simulink model "Q2"  (R2018a)
settings: Solver=VariableStepDiscrete  StartTime=0.0  StopTime=10  RelTol=1e-3
libraries: powerlib x10
settings Model: Creator=enes_  LastModifiedBy=nailt
settings CodeAppCC: StateflowObjectComments=on

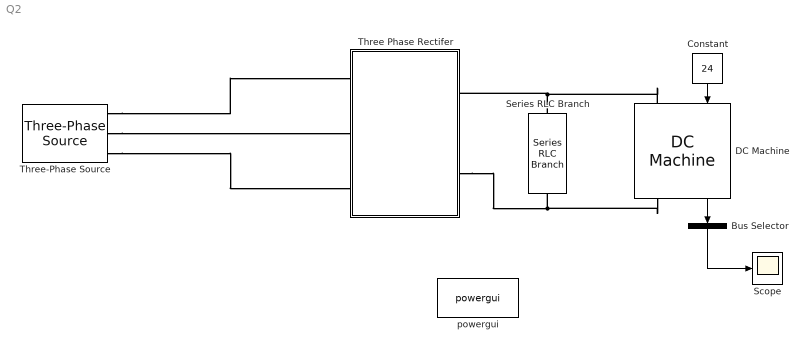
== system Q2 ==
  Bus Selector : BusSelector  OutputSignals=Armature current ia (A),Speed wm (rad/s),Electrical torque Te (n m)  OutputAsBus=on
  Constant : Constant  Value=24
  DC Machine : powerlib/Machines/DC Machine  PresetModel=No  MechanicalLoad=Torque TL  FieldType=Permanent magnet  ShowDetailedParameters=on  MeasurementBus=off  RLa="[10  0.01]"  RLf="[ 240  120]"  Laf=1.8  MachineConstant=Back-emf constant (V/rpm)  Ke=0.3  J=0.4  Bm=0  Tf=0  w0=1  Ifinit=1  TsPowergui=0  TsBlock=-1
  Scope : Scope
  Series RLC Branch : powerlib/Elements/Series RLC Branch  LConnTagsString=__new0  RConnTagsString=__new0  BranchType=C  Resistance=1  Inductance=1e-3  SetiL0=off  InitialCurrent=0  Capacitance=470e-6  Setx0=off  InitialVoltage=0  Measurements=None
  Three Phase Rectifer : Subsystem  AncestorBlock=halfcontrolled/Three Phase Rectifer
  Three-Phase Source : powerlib/Electrical Sources/Three-Phase Source  InternalConnection=Yg  VoltagePhases=off  Voltage=400  PhaseAngle=0  Voltage_phases=[25e3 25e3 25e3]/sqrt(3)  PhaseAngles_phases=[0 -120 +120]  Frequency=50  NonIdealSource=on  SpecifyImpedance=off  Resistance=100e-3  Inductance=100e-6  ShortCircuitLevel=100e6  BaseVoltage=400  XRratio=7  BusType=swing  Pref=10e3  Qref=0  Prefabc=[10e3, 10e3, 10e3]  Qrefabc=[0, 0, 0]  Qmin=-inf  Qmax=inf
  powergui : powerlib/powergui  Priority=1  SimulationMode=Discrete  SampleTime=50e-6  frequency=60  Iterations=50  frequencyindice=50  Pbase=100e6  ErrMax=1e-4  UnitsV=kV  UnitsW=MW  buscounter=0  FunctionMessages=off  echomessages=off  EnableUseOfTLC=off  CurrentSourceSwitches=off  DisableSnubberDevices=off  DisableRonSwitches=off  DisableVfSwitches=off  DisplayEquations=off  SolverType=Tustin/Backward Euler (TBE)  Interpol=off  ExternalGateDelay=off  methode=off  Ts=100  x0status=blocks  SPID=on  SwTol=0  HookPort=off  RestoreLinks=warning  ResistiveCurrentMeasurement=off  Frange=[0:2:500]  Ylog=off  Xlog=on  ShowGrid=off  save=off  variable=ZData  structure=0  ZoomFFT=off  StartTime=0.0  cycles=1  DisplayStyle=1  fundamental=60  FreqAxis=off  MaxFrequency=1000  frequencyindicesteady=1  RmsSteady=1  display=off
  wires:
  Constant/1 -> DC Machine/1
  DC Machine/1 -> Bus Selector/1
  Bus Selector/1 -> Scope/1
  connections:
  Three-Phase Source/RConn2 -- Three Phase Rectifer/LConn2
  Three-Phase Source/RConn1 -- Three Phase Rectifer/LConn1
  Three-Phase Source/RConn3 -- Three Phase Rectifer/LConn3
  Series RLC Branch/LConn1 -- DC Machine/LConn1 -- Three Phase Rectifer/RConn1
  Three Phase Rectifer/RConn2 -- DC Machine/RConn1 -- Series RLC Branch/RConn1

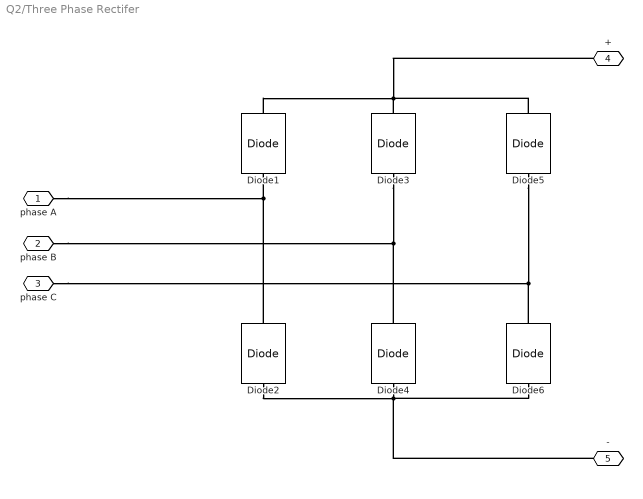
== system Q2/Three Phase Rectifer ==
  Diode{1..6} (6 alike) : powerlib/Power Electronics/Diode  Ron=0.02  Lon=0  Vf=0.8  IC=0  UseSnubber=0  Rs=10e9  Cs=250e-12  Measurements=off
  phase A : PMIOPort  Side=Left
  phase B : PMIOPort  Port=2  Side=Left
  phase C : PMIOPort  Port=3  Side=Left
  + : PMIOPort  Port=4  Side=Right
  - : PMIOPort  Port=5  Side=Right
  connections:
  phase C/RConn1 -- Diode5/LConn1 -- Diode6/RConn1
  phase A/RConn1 -- Diode2/RConn1 -- Diode1/LConn1
  Diode1/RConn1 -- Diode3/RConn1 -- Diode5/RConn1 -- +/RConn1
  phase B/RConn1 -- Diode3/LConn1 -- Diode4/RConn1
  -/RConn1 -- Diode6/LConn1 -- Diode4/LConn1 -- Diode2/LConn1
